simulink model "multirotor_full_system_psi0"  (R2023b)
settings: Solver=VariableStepAuto  StartTime=0.0  StopTime=100  RelTol=1e-3
values from neighbouring files (symbols this model uses):
  centre = [0;0;-3]    [run_quadcopter_sim.m]    (also in run_quadcopter_sim_psi0.m)
  omega = velocity/radius    (= 0.1)    [run_quadcopter_sim.m]    (also in run_quadcopter_sim_psi0.m)
  radius = 10    [run_quadcopter_sim.m]    (also in run_quadcopter_sim_psi0.m)
libraries: slpidlib x3
settings Model: Creator=yizho  LastModifiedBy=pouya

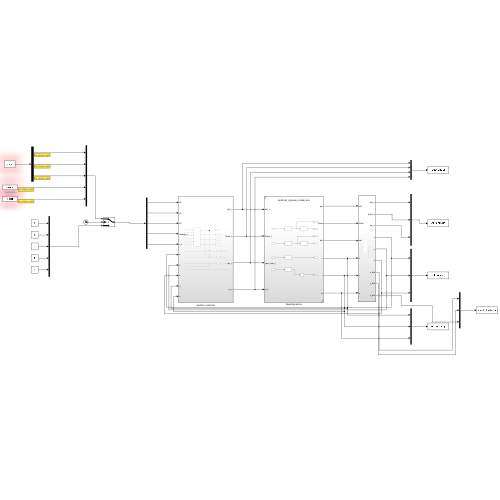
[thumbnail: Simulink's stored preview of the top-level diagram]
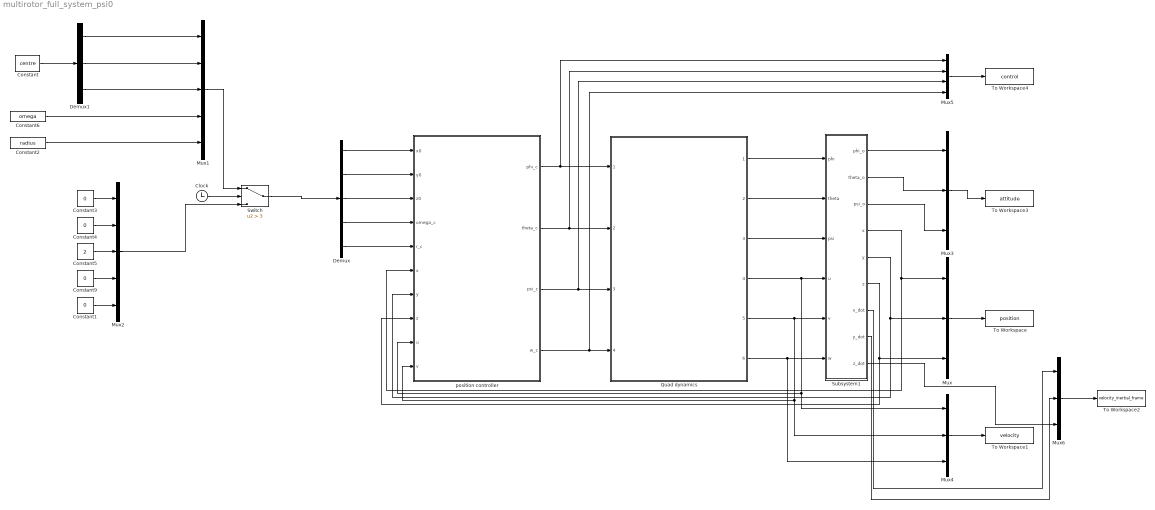
== system multirotor_full_system_psi0 ==
  Clock : Clock
  Constant : Constant  Value=centre
  Constant{1,3..4,9} (4 alike) : Constant  Value=0
  Constant2 : Constant  Value=radius
  Constant5 : Constant  Value=2
  Constant6 : Constant  Value=omega
  Demux : Demux  Outputs=5
  Demux1 : Demux  Outputs=3
  Mux{,3..4,6} (4 alike) : Mux  Inputs=3
  Mux1 : Mux  Inputs=5
  Mux2 : Mux  Inputs=5
  Mux5 : Mux
  Quad dynamics : Subsystem  ReferencedSubsystem=multirotor_dynamic_model_sim
  Subsystem1 : Subsystem
  Switch : Switch  Criteria=u2 > Threshold  Threshold=3  SaturateOnIntegerOverflow=off  InputSameDT=off
  To Workspace : ToWorkspace  VariableName=position  SaveFormat=Timeseries  SampleTime=-1
  To Workspace1 : ToWorkspace  VariableName=velocity  SaveFormat=Timeseries  SampleTime=-1
  To Workspace2 : ToWorkspace  VariableName=velocity_inertial_frame  SaveFormat=Timeseries  SampleTime=-1
  To Workspace3 : ToWorkspace  VariableName=attitude  SaveFormat=Timeseries  SampleTime=-1
  To Workspace4 : ToWorkspace  VariableName=control  SaveFormat=Timeseries  SampleTime=-1
  position controller : Subsystem
  wires:
  Mux4/1 -> To Workspace1/1
  Mux/1 -> To Workspace/1
  position controller/2(theta_c) -> Mux5/2, Quad dynamics/2
  Constant4/1 -> Mux2/2
  position controller/4(w_c) -> Mux5/4, Quad dynamics/4
  position controller/1(phi_c) -> Mux5/1, Quad dynamics/1
  Demux/1 -> position controller/1(x0)
  Constant1/1 -> Mux2/5
  Demux/3 -> position controller/3(z0)
  Clock/1 -> Switch/2
  Constant3/1 -> Mux2/1
  Mux3/1 -> To Workspace3/1
  Demux/2 -> position controller/2(y0)
  Constant5/1 -> Mux2/3
  position controller/3(psi_c) -> Mux5/3, Quad dynamics/3
  Constant9/1 -> Mux2/4
  Mux5/1 -> To Workspace4/1
  Mux2/1 -> Switch/3
  Quad dynamics/1 -> Subsystem1/1(phi)
  Quad dynamics/2 -> Subsystem1/2(theta)
  Quad dynamics/4 -> Mux4/1, position controller/9(u), Subsystem1/4(u)
  Quad dynamics/5 -> Mux4/2, position controller/10(v), Subsystem1/5(v)
  Quad dynamics/6 -> Mux4/3, Subsystem1/6(w)
  Subsystem1/5(y) -> Mux/2, position controller/7(y)
  Subsystem1/4(x) -> Mux/1, position controller/6(x)
  Quad dynamics/3 -> Subsystem1/3(psi)
  Subsystem1/3(psi_o) -> Mux3/3
  Subsystem1/2(theta_o) -> Mux3/2
  Subsystem1/1(phi_o) -> Mux3/1
  Subsystem1/6(z) -> Mux/3, position controller/8(z)
  Demux/4 -> position controller/4(omega_c)
  Demux/5 -> position controller/5(r_c)
  Mux6/1 -> To Workspace2/1
  Subsystem1/7(x_dot) -> Mux6/1
  Subsystem1/8(y_dot) -> Mux6/2
  Subsystem1/9(z_dot) -> Mux6/3
  Constant/1 -> Demux1/1
  Demux1/3 -> Mux1/3
  Demux1/2 -> Mux1/2
  Demux1/1 -> Mux1/1
  Constant6/1 -> Mux1/4
  Constant2/1 -> Mux1/5
  Switch/1 -> Demux/1
  Mux1/1 -> Switch/1

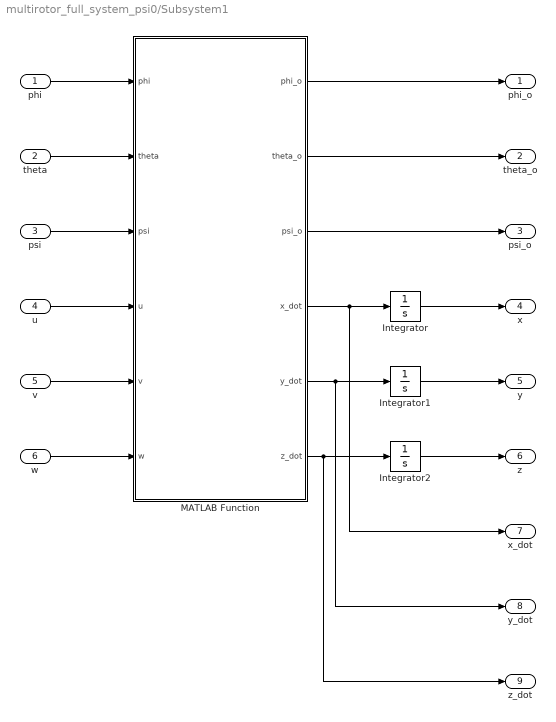
== system multirotor_full_system_psi0/Subsystem1 ==
  phi : Inport
  theta : Inport  Port=2
  psi : Inport  Port=3
  u : Inport  Port=4
  v : Inport  Port=5
  w : Inport  Port=6
  Integrator : Integrator
  Integrator1 : Integrator
  Integrator2 : Integrator
  MATLAB Function : MATLAB Function  TreatAsAtomicUnit=on
  phi_o : Outport
  theta_o : Outport  Port=2
  psi_o : Outport  Port=3
  x : Outport  Port=4
  y : Outport  Port=5
  z : Outport  Port=6
  x_dot : Outport  Port=7
  y_dot : Outport  Port=8
  z_dot : Outport  Port=9
  wires:
  phi/1 -> MATLAB Function/1(phi)
  psi/1 -> MATLAB Function/3(psi)
  theta/1 -> MATLAB Function/2(theta)
  MATLAB Function/6(z_dot) -> z_dot/1, Integrator2/1
  MATLAB Function/4(x_dot) -> x_dot/1, Integrator/1
  MATLAB Function/5(y_dot) -> y_dot/1, Integrator1/1
  Integrator/1 -> x/1
  Integrator1/1 -> y/1
  Integrator2/1 -> z/1
  u/1 -> MATLAB Function/4(u)
  v/1 -> MATLAB Function/5(v)
  w/1 -> MATLAB Function/6(w)
  MATLAB Function/3(psi_o) -> psi_o/1
  MATLAB Function/2(theta_o) -> theta_o/1
  MATLAB Function/1(phi_o) -> phi_o/1

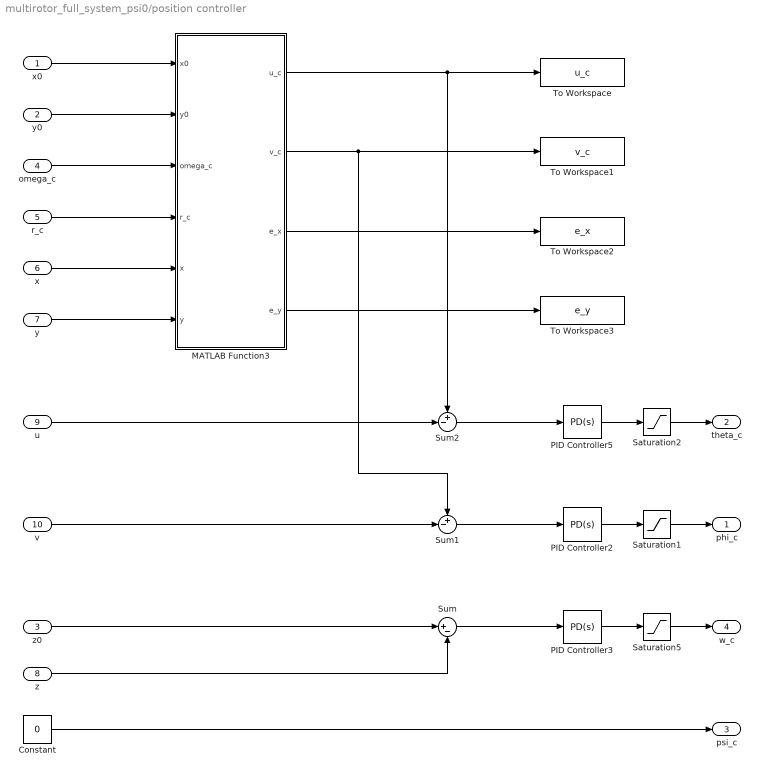
== system multirotor_full_system_psi0/position controller ==
  x0 : Inport
  y0 : Inport  Port=2
  z0 : Inport  Port=3
  omega_c : Inport  Port=4
  r_c : Inport  Port=5
  x : Inport  Port=6
  y : Inport  Port=7
  z : Inport  Port=8
  u : Inport  Port=9
  v : Inport  Port=10
  Constant : Constant  Value=0
  MATLAB Function3 : MATLAB Function  TreatAsAtomicUnit=on
  PID Controller2 : slpidlib/PID Controller  Controller=PD  Form=Parallel  TimeDomain=Continuous-time  UseExternalTs=off  SampleTime=-1  IntegratorMethod=Forward Euler  FilterMethod=Forward Euler  ControllerParametersSource=internal  P=2.94092069866743  I=-0.000905529611353649  UseKiTs=off  D=0.489137008553763  N=147.769658124209  UseFilter=on  TunerSelectOption=Transfer Function Based (PID Tuner App)  InitialConditionSource=internal  InitialConditionForIntegrator=0  InitialConditionForFilter=0  DifferentiatorICPrevScaledInput=0  ExternalReset=none  TrackingMode=off  Kt=1  LimitOutput=off  SatLimitsSource=internal  UpperSaturationLimit=inf  LowerSaturationLimit=-inf  LinearizeAsGain=on  AntiWindupMode=none  Kb=1  LimitIntegrator=off  UpperIntegratorSaturationLimit=inf  LowerIntegratorSaturationLimit=-inf  POutMin=[]  POutMax=[]  IOutMin=[]  IOutMax=[]  DOutMin=[]  DOutMax=[]  NOutMin=[]  NOutMax=[]  SumOutMin=[]  SumOutMax=[]  SaturationOutMin=[]  SaturationOutMax=[]  PParamMin=[]  PParamMax=[]  IParamMin=[]  IParamMax=[]  DParamMin=[]  DParamMax=[]  NParamMin=[]  NParamMax=[]  KbParamMin=[]  KbParamMax=[]  KtParamMin=[]  KtParamMax=[]  KbOutMin=[]  KbOutMax=[]  KtOutMin=[]  KtOutMax=[]  IntegratorOutMin=[]  IntegratorOutMax=[]  FilterOutMin=[]  FilterOutMax=[]  SumI1OutMin=[]  SumI1OutMax=[]  SumI2OutMin=[]  SumI2OutMax=[]  SumI3OutMin=[]  SumI3OutMax=[]  SumI4OutMin=[]  SumI4OutMax=[]  SumDOutMin=[]  SumDOutMax=[]  DifferentiatorOutMin=[]  DifferentiatorOutMax=[]  FilterDiffOutCoefMin=[]  FilterDiffOutCoefMax=[]  ReciprocalOutMin=[]  ReciprocalOutMax=[]  SumDenOutMin=[]  SumDenOutMax=[]  SumNumOutMin=[]  SumNumOutMax=[]  DivideOutMin=[]  DivideOutMax=[]  UdiffTsProdOutMin=[]  UdiffTsProdOutMax=[]  NTsProdOutMin=[]  NTsProdOutMax=[]  UintegralTsProdOutMin=[]  UintegralTsProdOutMax=[]  UngainTsProdOutMin=[]  UngainTsProdOutMax=[]  ClampingZeroOutDataTypeStr=Inherit: Inherit via back propagation  ClampingZeroOutMin=[]  ClampingZeroOutMax=[]  FilterDenConstantOutDataTypeStr=Inherit: Inherit via back propagation  FilterDenConstantOutMin=[]  FilterDenConstantOutMax=[]  PCopyOutDataTypeStr=Inherit: Inherit via back propagation  PCopyOutMin=[]  PCopyOutMax=[]  NCopyOutDataTypeStr=Inherit: Inherit via back propagation  NCopyOutMin=[]  NCopyOutMax=[]  IntegratorContinuousStateAttributes=''  IntegratorStateMustResolveToSignalObject=off  IntegratorRTWStateStorageClass=Auto  FilterContinuousStateAttributes=''  FilterStateMustResolveToSignalObject=off  FilterRTWStateStorageClass=Auto  ParallelPVariant=InternalParameters  IdealPVariant=Disabled  IVariant=Disabled  DVariant=InternalParameters  IntegratorVariant=Disabled  SatVariant=Disabled  AWVariant=Disabled  PCopyVariant=Disabled  TRVariant=Disabled  FdbkBlocksVariant=Forward  IdealPFdbkVariant=Disabled  SatFdbkVariant=Disabled  DerivativeFilterVariant=ContFilter  NVariant=InternalParameters  NCopyVariant=Disabled  FilterICVariant=InternalICsFilter  IntegratorICVariant=Disabled  ExternalResetVariant=Disabled  TRSumVariant=Passthrough  SumFdbkVariant=Disabled  SumVariant=Sum_PD  TsampFilterVariant=InternalTs  TsampNgainVariant=Passthrough  TsampIntegralVariant=Disabled_SignalSpec  ExternalSaturationOutDataTypeStr=Inherit: Same as second input
  PID Controller3 : slpidlib/PID Controller  Controller=PD  Form=Parallel  TimeDomain=Continuous-time  UseExternalTs=off  SampleTime=-1  IntegratorMethod=Forward Euler  FilterMethod=Forward Euler  ControllerParametersSource=internal  P=8.1174906201866  I=0.001  UseKiTs=off  D=2  N=28.4037357731719  UseFilter=on  TunerSelectOption=Transfer Function Based (PID Tuner App)  InitialConditionSource=internal  InitialConditionForIntegrator=0  InitialConditionForFilter=0  DifferentiatorICPrevScaledInput=0  ExternalReset=none  TrackingMode=off  Kt=1  LimitOutput=off  SatLimitsSource=internal  UpperSaturationLimit=inf  LowerSaturationLimit=-inf  LinearizeAsGain=on  AntiWindupMode=none  Kb=1  LimitIntegrator=off  UpperIntegratorSaturationLimit=inf  LowerIntegratorSaturationLimit=-inf  POutMin=[]  POutMax=[]  IOutMin=[]  IOutMax=[]  DOutMin=[]  DOutMax=[]  NOutMin=[]  NOutMax=[]  SumOutMin=[]  SumOutMax=[]  SaturationOutMin=[]  SaturationOutMax=[]  PParamMin=[]  PParamMax=[]  IParamMin=[]  IParamMax=[]  DParamMin=[]  DParamMax=[]  NParamMin=[]  NParamMax=[]  KbParamMin=[]  KbParamMax=[]  KtParamMin=[]  KtParamMax=[]  KbOutMin=[]  KbOutMax=[]  KtOutMin=[]  KtOutMax=[]  IntegratorOutMin=[]  IntegratorOutMax=[]  FilterOutMin=[]  FilterOutMax=[]  SumI1OutMin=[]  SumI1OutMax=[]  SumI2OutMin=[]  SumI2OutMax=[]  SumI3OutMin=[]  SumI3OutMax=[]  SumI4OutMin=[]  SumI4OutMax=[]  SumDOutMin=[]  SumDOutMax=[]  DifferentiatorOutMin=[]  DifferentiatorOutMax=[]  FilterDiffOutCoefMin=[]  FilterDiffOutCoefMax=[]  ReciprocalOutMin=[]  ReciprocalOutMax=[]  SumDenOutMin=[]  SumDenOutMax=[]  SumNumOutMin=[]  SumNumOutMax=[]  DivideOutMin=[]  DivideOutMax=[]  UdiffTsProdOutMin=[]  UdiffTsProdOutMax=[]  NTsProdOutMin=[]  NTsProdOutMax=[]  UintegralTsProdOutMin=[]  UintegralTsProdOutMax=[]  UngainTsProdOutMin=[]  UngainTsProdOutMax=[]  ClampingZeroOutDataTypeStr=Inherit: Inherit via back propagation  ClampingZeroOutMin=[]  ClampingZeroOutMax=[]  FilterDenConstantOutDataTypeStr=Inherit: Inherit via back propagation  FilterDenConstantOutMin=[]  FilterDenConstantOutMax=[]  PCopyOutDataTypeStr=Inherit: Inherit via back propagation  PCopyOutMin=[]  PCopyOutMax=[]  NCopyOutDataTypeStr=Inherit: Inherit via back propagation  NCopyOutMin=[]  NCopyOutMax=[]  IntegratorContinuousStateAttributes=''  IntegratorStateMustResolveToSignalObject=off  IntegratorRTWStateStorageClass=Auto  FilterContinuousStateAttributes=''  FilterStateMustResolveToSignalObject=off  FilterRTWStateStorageClass=Auto  ParallelPVariant=InternalParameters  IdealPVariant=Disabled  IVariant=Disabled  DVariant=InternalParameters  IntegratorVariant=Disabled  SatVariant=Disabled  AWVariant=Disabled  PCopyVariant=Disabled  TRVariant=Disabled  FdbkBlocksVariant=Forward  IdealPFdbkVariant=Disabled  SatFdbkVariant=Disabled  DerivativeFilterVariant=ContFilter  NVariant=InternalParameters  NCopyVariant=Disabled  FilterICVariant=InternalICsFilter  IntegratorICVariant=Disabled  ExternalResetVariant=Disabled  TRSumVariant=Passthrough  SumFdbkVariant=Disabled  SumVariant=Sum_PD  TsampFilterVariant=InternalTs  TsampNgainVariant=Passthrough  TsampIntegralVariant=Disabled_SignalSpec  ExternalSaturationOutDataTypeStr=Inherit: Same as second input
  PID Controller5 : slpidlib/PID Controller  Controller=PD  Form=Parallel  TimeDomain=Continuous-time  UseExternalTs=off  SampleTime=-1  IntegratorMethod=Forward Euler  FilterMethod=Forward Euler  ControllerParametersSource=internal  P=-2.34944256970404  I=-0.001  UseKiTs=off  D=-0.490714659968128  N=94.7705767439824  UseFilter=on  TunerSelectOption=Transfer Function Based (PID Tuner App)  InitialConditionSource=internal  InitialConditionForIntegrator=0  InitialConditionForFilter=0  DifferentiatorICPrevScaledInput=0  ExternalReset=none  TrackingMode=off  Kt=1  LimitOutput=off  SatLimitsSource=internal  UpperSaturationLimit=inf  LowerSaturationLimit=-inf  LinearizeAsGain=on  AntiWindupMode=none  Kb=1  LimitIntegrator=off  UpperIntegratorSaturationLimit=inf  LowerIntegratorSaturationLimit=-inf  POutMin=[]  POutMax=[]  IOutMin=[]  IOutMax=[]  DOutMin=[]  DOutMax=[]  NOutMin=[]  NOutMax=[]  SumOutMin=[]  SumOutMax=[]  SaturationOutMin=[]  SaturationOutMax=[]  PParamMin=[]  PParamMax=[]  IParamMin=[]  IParamMax=[]  DParamMin=[]  DParamMax=[]  NParamMin=[]  NParamMax=[]  KbParamMin=[]  KbParamMax=[]  KtParamMin=[]  KtParamMax=[]  KbOutMin=[]  KbOutMax=[]  KtOutMin=[]  KtOutMax=[]  IntegratorOutMin=[]  IntegratorOutMax=[]  FilterOutMin=[]  FilterOutMax=[]  SumI1OutMin=[]  SumI1OutMax=[]  SumI2OutMin=[]  SumI2OutMax=[]  SumI3OutMin=[]  SumI3OutMax=[]  SumI4OutMin=[]  SumI4OutMax=[]  SumDOutMin=[]  SumDOutMax=[]  DifferentiatorOutMin=[]  DifferentiatorOutMax=[]  FilterDiffOutCoefMin=[]  FilterDiffOutCoefMax=[]  ReciprocalOutMin=[]  ReciprocalOutMax=[]  SumDenOutMin=[]  SumDenOutMax=[]  SumNumOutMin=[]  SumNumOutMax=[]  DivideOutMin=[]  DivideOutMax=[]  UdiffTsProdOutMin=[]  UdiffTsProdOutMax=[]  NTsProdOutMin=[]  NTsProdOutMax=[]  UintegralTsProdOutMin=[]  UintegralTsProdOutMax=[]  UngainTsProdOutMin=[]  UngainTsProdOutMax=[]  ClampingZeroOutDataTypeStr=Inherit: Inherit via back propagation  ClampingZeroOutMin=[]  ClampingZeroOutMax=[]  FilterDenConstantOutDataTypeStr=Inherit: Inherit via back propagation  FilterDenConstantOutMin=[]  FilterDenConstantOutMax=[]  PCopyOutDataTypeStr=Inherit: Inherit via back propagation  PCopyOutMin=[]  PCopyOutMax=[]  NCopyOutDataTypeStr=Inherit: Inherit via back propagation  NCopyOutMin=[]  NCopyOutMax=[]  IntegratorContinuousStateAttributes=''  IntegratorStateMustResolveToSignalObject=off  IntegratorRTWStateStorageClass=Auto  FilterContinuousStateAttributes=''  FilterStateMustResolveToSignalObject=off  FilterRTWStateStorageClass=Auto  ParallelPVariant=InternalParameters  IdealPVariant=Disabled  IVariant=Disabled  DVariant=InternalParameters  IntegratorVariant=Disabled  SatVariant=Disabled  AWVariant=Disabled  PCopyVariant=Disabled  TRVariant=Disabled  FdbkBlocksVariant=Forward  IdealPFdbkVariant=Disabled  SatFdbkVariant=Disabled  DerivativeFilterVariant=ContFilter  NVariant=InternalParameters  NCopyVariant=Disabled  FilterICVariant=InternalICsFilter  IntegratorICVariant=Disabled  ExternalResetVariant=Disabled  TRSumVariant=Passthrough  SumFdbkVariant=Disabled  SumVariant=Sum_PD  TsampFilterVariant=InternalTs  TsampNgainVariant=Passthrough  TsampIntegralVariant=Disabled_SignalSpec  ExternalSaturationOutDataTypeStr=Inherit: Same as second input
  Saturation1 : Saturate  UpperLimit=1  LowerLimit=-1
  Saturation2 : Saturate  UpperLimit=1  LowerLimit=-1
  Saturation5 : Saturate  UpperLimit=1  LowerLimit=-1
  Sum : Sum  Inputs=|+-
  Sum1 : Sum  Inputs=+-|
  Sum2 : Sum  Inputs=+-|
  To Workspace : ToWorkspace  VariableName=u_c  SaveFormat=Timeseries  SampleTime=-1
  To Workspace1 : ToWorkspace  VariableName=v_c  SaveFormat=Timeseries  SampleTime=-1
  To Workspace2 : ToWorkspace  VariableName=e_x  SaveFormat=Timeseries  SampleTime=-1
  To Workspace3 : ToWorkspace  VariableName=e_y  SaveFormat=Timeseries  SampleTime=-1
  phi_c : Outport
  theta_c : Outport  Port=2
  psi_c : Outport  Port=3
  w_c : Outport  Port=4
  wires:
  Saturation1/1 -> phi_c/1
  Saturation2/1 -> theta_c/1
  Saturation5/1 -> w_c/1
  Constant/1 -> psi_c/1
  x0/1 -> MATLAB Function3/1(x0)
  y0/1 -> MATLAB Function3/2(y0)
  x/1 -> MATLAB Function3/5(x)
  y/1 -> MATLAB Function3/6(y)
  omega_c/1 -> MATLAB Function3/3(omega_c)
  r_c/1 -> MATLAB Function3/4(r_c)
  z/1 -> Sum/2
  z0/1 -> Sum/1
  PID Controller2/1 -> Saturation1/1
  PID Controller5/1 -> Saturation2/1
  u/1 -> Sum2/2
  v/1 -> Sum1/2
  MATLAB Function3/2(v_c) -> Sum1/1, To Workspace1/1
  MATLAB Function3/1(u_c) -> Sum2/1, To Workspace/1
  PID Controller3/1 -> Saturation5/1
  Sum2/1 -> PID Controller5/1
  Sum1/1 -> PID Controller2/1
  Sum/1 -> PID Controller3/1
  MATLAB Function3/3(e_x) -> To Workspace2/1
  MATLAB Function3/4(e_y) -> To Workspace3/1

== matlab function multirotor_full_system_psi0/Subsystem1/MATLAB Function ==
  data: phi_o output; theta_o output; psi_o output; phi input; theta input; psi input; x_dot output; y_dot output; u input; v input; w input; z_dot output
function [phi_o, theta_o, psi_o, x_dot, y_dot, z_dot] = fcn(phi, theta, psi, u, v, w)

% s1 = sin(phi);
% c1 = cos(phi);
% s2 = sin(theta);
% c2 = cos(theta);
% s3 = sin(psi);
% c3 = cos(psi);

% s1 = 0;
% c1 = 1;
% s2 = 0;
% c2 = 1;
% s3 = sin(psi);
% c3 = cos(psi);

% x_dot = u * (c2 * c3) + v * (s1 * s2 * c3 - c1 * s3) + w * (c1 * s2 * c3 + s1 * s3);
% y_dot = u * (c2 * s3) + v * (s1 * s2 * s3 - c1 * c3) + w * (c1 * s2 * s3 - s1 * c3);
% z_dot = u * (-s2) + v * s1 * c2 + w * c1 * c2;

x_dot = u;
y_dot = v;
z_dot = w;

phi_o = phi;
theta_o = theta;
psi_o = psi;

== matlab function multirotor_full_system_psi0/position controller/MATLAB Function3 ==
  data: x0 input; u_c output; y0 input; omega_c input; r_c input; x input; y input; v_c output; e_x output; e_y output
function [u_c, v_c, e_x, e_y] = calc_reference(x0, y0, omega_c, r_c, x, y)

speed = omega_c * r_c;

dx = x - x0;
dy = y - y0;
gamma = atan2(dy, dx); % direction to center (or tracked position if r = 0)

x_c = x0 + r_c * cos(gamma);
y_c = y0 + r_c * sin(gamma);

e_x = x_c - x;
e_y = y_c - y;

beta = gamma + pi / 2; % * omega_c / abs(omega_c); % direction of orbiting velocity
u_c = speed * cos(beta) + e_x;
v_c = speed * sin(beta) + e_y;

k = 1;
